simulink model "sm_tVtest_roller_idlerArm_i2u0l3"  (R2026a)
settings: Solver=VariableStepAuto  AbsTol=1e-3  EnableMultiTasking=on
undefined symbols (not defined in the file): P1, P2, P3, P4, P5, X, Y, Z
libraries: sm_lib x5, sm_trackV_lib_terrain_contact_elem x5, fl_lib x2, nesl_utility x2, sm_trackV_lib_chain_underc_elem x1, simulink x1, sm_rollerV_lib_underc_elem x1, sm_rollerV_lib_underc_idlerArm_i2u0l3 x1
Description:
  | Copyright 2024-2026 The MathWorks, Inc.
settings Model: Creator=smiller  LastModifiedBy=smiller
settings DebuggingCC: SubsystemReferenceDiagnosticForUnitTest=warning
settings SimscapeCC: SimscapeNominalValues="[{\"value\":\"1\",\"unit\":\"A\"},{\"value\":\"1\",\"unit\":\"bar\"},{\"value\":\"1\",\"unit\":\"cm^2\"},{\"value\":\"1\",\"unit\":\"cm^3/s\"},{\"value\":\"1\",\"unit\":\"kJ/kg\"},{\"value\":\"1\",\"unit\":\"kW\"},{\"value\":\"1\",\"unit\":\"l\"},{\"value\":\"1\",\"unit\":\"N\"},{\"value\":\"1\",\"unit\":\"N*m\"},{\"value\":\"1\",\"unit\":\"V\"}]"  SimscapeLogSimulationStatistics=on
settings DiagnosticsConfigSet: SimMechanicsUnconnectedFramePorts=none
settings ExplorerConfigSet: InternalSimMechanicsExplorerSettings="<ExplorerConfiguration><canonicalview>default</canonicalview><AnimationSetting><BasePlaybackSpeed>1.0</BasePlaybackSpeed><PlaybackSpeedFactor>1.0</PlaybackSpeedFactor></AnimationSetting><TilePanel><TileInfo><Tiles Columns=\"1\" Count=\"1\" Rows=\"1\"><Column Weight=\"1\"/><Row Weight=\"1\"/><Tile Height=\"1\" Width=\"1\" X=\"0\" Y=\"0\"/></Tiles></TileInfo><SceneInfo><SceneViewer><BGColor><R>1</R><G>1</G><B>1</B></BGColor><Camera><DoPerspective>off</DoPerspective><Position><X>0.567898563386482147</X><Y>-1.86694805060514923</Y><Z>1.30068286552298851</Z></Position><Center><X>0.185623686788384534</X><Y>-0.0132287901313050682</Y><Z>1.03548068078574151</Z></Center><Up><X>-0.02328869963817011</X><Y>0.136876623335939085</Y><Z>0.990314306901255881</Z></Up><ViewLimDist>1</ViewLimDist><YLim>1.16506449341773988</YLim><XLim>2.52473886880948983</XLim></Camera></SceneViewer></SceneInfo></TilePanel><MechEditorPanel><Cameras/><GfxPanelCameraMap/><VideoCreator><PlaybackSpeedRatio>1.0</PlaybackSpeedRatio><FrameRate>30</FrameRate><VideoFormat>Motion JPEG AVI</VideoFormat><FrameSize>auto</FrameSize></VideoCreator></MechEditorPanel></ExplorerConfiguration>"

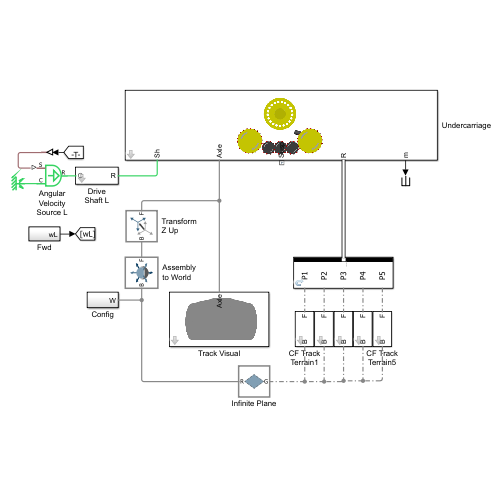
[thumbnail: Simulink's stored preview of the top-level diagram]
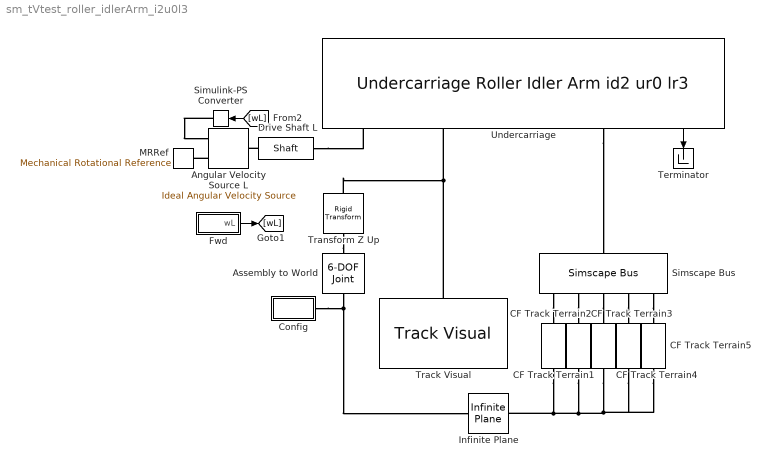
== system sm_tVtest_roller_idlerArm_i2u0l3 ==
  Angular Velocity Source L : fl_lib/Mechanical/Mechanical Sources/Ideal Angular Velocity Source
  Assembly to World : sm_lib/Joints/6-DOF Joint  JointMode=Normal  CompositeWrenchDir=FollowerOnBase  CompositeWrenchFrame=BaseFrame  SenseConstraintForce=off  SenseConstraintTorque=off  SenseTotalForce=off  SenseTotalTorque=off  PxPositionTargetSpecify=off  PxPositionTargetPriority=High  PxPositionTargetValue=0  PxPositionTargetValueUnits=m  PxVelocityTargetSpecify=off  PxVelocityTargetPriority=High  PxVelocityTargetValue=0  PxVelocityTargetValueUnits=m/s  PxEquilibriumPosition=0  PxEquilibriumPositionUnits=m  PxSpringStiffness=0  PxSpringStiffnessUnits=N/m  PxDampingCoefficient=0  PxDampingCoefficientUnits=N/(m/s)  PxLowerLimitSpecify=off  PxLowerLimitBound=-1  PxLowerLimitBoundUnits=m  PxLowerLimitStiffness=1e6  PxLowerLimitStiffnessUnits=N/m  PxLowerLimitDamping=1e3  PxLowerLimitDampingUnits=N/(m/s)  PxLowerLimitTransitionRegionWidth=1e-4  PxLowerLimitTransitionRegionWidthUnits=m  PxUpperLimitSpecify=off  PxUpperLimitBound=1  PxUpperLimitBoundUnits=m  PxUpperLimitStiffness=1e6  PxUpperLimitStiffnessUnits=N/m  PxUpperLimitDamping=1e3  PxUpperLimitDampingUnits=N/(m/s)  PxUpperLimitTransitionRegionWidth=1e-4  PxUpperLimitTransitionRegionWidthUnits=m  PxTorqueActuationMode=NoTorque  PxMotionActuationMode=ComputedMotion  PxSensePosition=off  PxSenseVelocity=off  PxSenseAcceleration=off  PxSenseTorqueForce=off  PxSenseLowerLimitTorqueForce=off  PxSenseUpperLimitTorqueForce=off  PyPositionTargetSpecify=off  PyPositionTargetPriority=High  PyPositionTargetValue=0  PyPositionTargetValueUnits=m  PyVelocityTargetSpecify=off  PyVelocityTargetPriority=High  PyVelocityTargetValue=0  PyVelocityTargetValueUnits=m/s  PyEquilibriumPosition=0  PyEquilibriumPositionUnits=m  PySpringStiffness=0  PySpringStiffnessUnits=N/m  PyDampingCoefficient=0  PyDampingCoefficientUnits=N/(m/s)  PyLowerLimitSpecify=off  PyLowerLimitBound=-1  PyLowerLimitBoundUnits=m  PyLowerLimitStiffness=1e6  PyLowerLimitStiffnessUnits=N/m  PyLowerLimitDamping=1e3  PyLowerLimitDampingUnits=N/(m/s)  PyLowerLimitTransitionRegionWidth=1e-4  PyLowerLimitTransitionRegionWidthUnits=m  PyUpperLimitSpecify=off  PyUpperLimitBound=1  PyUpperLimitBoundUnits=m  PyUpperLimitStiffness=1e6  PyUpperLimitStiffnessUnits=N/m  PyUpperLimitDamping=1e3  PyUpperLimitDampingUnits=N/(m/s)  PyUpperLimitTransitionRegionWidth=1e-4  PyUpperLimitTransitionRegionWidthUnits=m  PyTorqueActuationMode=NoTorque  PyMotionActuationMode=ComputedMotion  PySensePosition=off  PySenseVelocity=off  PySenseAcceleration=off  PySenseTorqueForce=off  PySenseLowerLimitTorqueForce=off  PySenseUpperLimitTorqueForce=off  PzPositionTargetSpecify=on  PzPositionTargetPriority=High  PzPositionTargetValue=1.5  PzPositionTargetValueUnits=m  PzVelocityTargetSpecify=off  PzVelocityTargetPriority=High  PzVelocityTargetValue=0  PzVelocityTargetValueUnits=m/s  PzEquilibriumPosition=0  PzEquilibriumPositionUnits=m  PzSpringStiffness=0  PzSpringStiffnessUnits=N/m  PzDampingCoefficient=0  PzDampingCoefficientUnits=N/(m/s)  PzLowerLimitSpecify=off  PzLowerLimitBound=-1  PzLowerLimitBoundUnits=m  PzLowerLimitStiffness=1e6  PzLowerLimitStiffnessUnits=N/m  PzLowerLimitDamping=1e3  PzLowerLimitDampingUnits=N/(m/s)  PzLowerLimitTransitionRegionWidth=1e-4  PzLowerLimitTransitionRegionWidthUnits=m  PzUpperLimitSpecify=off  PzUpperLimitBound=1  PzUpperLimitBoundUnits=m  PzUpperLimitStiffness=1e6  PzUpperLimitStiffnessUnits=N/m  PzUpperLimitDamping=1e3  PzUpperLimitDampingUnits=N/(m/s)  PzUpperLimitTransitionRegionWidth=1e-4  PzUpperLimitTransitionRegionWidthUnits=m  PzTorqueActuationMode=NoTorque  PzMotionActuationMode=ComputedMotion  PzSensePosition=off  PzSenseVelocity=off  PzSenseAcceleration=off  PzSenseTorqueForce=off  PzSenseLowerLimitTorqueForce=off  PzSenseUpperLimitTorqueForce=off  SphPositionTargetSpecify=off  SphPositionTargetPriority=High  SphPositionTargetRotationMethod=None  SphPositionTargetFollAlignAxisA=+X  SphPositionTargetBaseAlignAxisA=+Y  SphPositionTargetFollAlignAxisB=+Y  SphPositionTargetBaseAlignAxisB=+Z  SphPositionTargetRotationStandardAxis=+Z  SphPositionTargetRotationAngle=0.0  SphPositionTargetRotationAngleUnits=deg  SphPositionTargetRotationArbitraryAxis=[0 0 1]  SphPositionTargetRotationSequenceAxes=FollowerAxes  SphPositionTargetRotationSequence=XYX  SphPositionTargetRotationSequenceAngles=[0 0 0]  SphPositionTargetRotationSequenceAnglesUnits=deg  SphPositionTargetRotationMatrix=[1 0 0; 0 1 0; 0 0 1]  SphPositionTargetQuaternion=[1 0 0 0]  SphVelocityTargetSpecify=off  SphVelocityTargetPriority=High  SphVelocityTargetValue=[0 0 0]  SphVelocityTargetValueUnits=deg/s  SphVelocityTargetInFollowerFrame=on  SphEqPosRotationMethod=None  SphEqPosFollAlignAxisA=+X  SphEqPosBaseAlignAxisA=+Y  SphEqPosFollAlignAxisB=+Y  SphEqPosBaseAlignAxisB=+Z  SphEqPosRotationStandardAxis=+Z  SphEqPosRotationAngle=0.0  SphEqPosRotationAngleUnits=deg  SphEqPosRotationArbitraryAxis=[0 0 1]  SphEqPosRotationSequenceAxes=FollowerAxes  SphEqPosRotationSequence=XYX  SphEqPosRotationSequenceAngles=[0 0 0]  SphEqPosRotationSequenceAnglesUnits=deg  SphEqPosRotationMatrix=[1 0 0; 0 1 0; 0 0 1]  SphEqPosQuaternion=[1 0 0 0]  SphSpringStiffness=0  SphSpringStiffnessUnits=N*m/deg  SphDampingCoefficient=0  SphDampingCoefficientUnits=N*m/(deg/s)  SphLowerLimitSpecify=off  SphLowerLimitBound=15  SphLowerLimitBoundUnits=deg  SphLowerLimitStiffness=1e4  SphLowerLimitStiffnessUnits=N*m/deg  SphLowerLimitDamping=10  SphLowerLimitDampingUnits=N*m/(deg/s)  SphLowerLimitTransitionRegionWidth=0.1  SphLowerLimitTransitionRegionWidthUnits=deg  SphUpperLimitSpecify=off  SphUpperLimitBound=45  SphUpperLimitBoundUnits=deg  SphUpperLimitStiffness=1e4  SphUpperLimitStiffnessUnits=N*m/deg  SphUpperLimitDamping=10  SphUpperLimitDampingUnits=N*m/(deg/s)  SphUpperLimitTransitionRegionWidth=0.1  SphUpperLimitTransitionRegionWidthUnits=deg  SphTorqueActuationMode=NoTorque  SphActuateTorqueX=off  SphActuateTorqueY=off  SphActuateTorqueZ=off  SphActuateTorque=off  SphActuationFrame=BaseFrame  SphSensePosition=off  SphSenseVelocityX=off  SphSenseVelocityY=off  SphSenseVelocityZ=off  SphSenseVelocity=off  SphSenseAccelerationX=off  SphSenseAccelerationY=off  SphSenseAccelerationZ=off  SphSenseAcceleration=off  SphSenseLowerLimitTorqueMag=off  SphSenseUpperLimitTorqueMag=off  SphSensingFrame=BaseFrame
  CF Track Terrain{1..5} (5 alike) : sm_trackV_lib_terrain_contact_elem/CF Track Terrain  NormalStiffness=Scene.Contact.Terrain.K  NormalDamping=Scene.Contact.Terrain.B  NormalTransitionRegionWidth=Scene.Contact.Terrain.TW  CoefficientOfDynamicFriction=Scene.Contact.Terrain.mud  CoefficientOfStaticFriction=Scene.Contact.Terrain.mus  FrictionalCriticalVelocity=Scene.Contact.Terrain.CV
  Config : Subsystem
  Drive Shaft L : sm_trackV_lib_chain_underc_elem/Shaft  k_shaft=Excv.Drive.Shaft.k  b_shaft=Excv.Drive.Shaft.b
  Fwd : Subsystem  VariantControl=Fwd
  Infinite Plane : sm_lib/Curves and Surfaces/Infinite Plane  GraphicType=Rectangle  GraphicPlaneWidth=1  GraphicPlaneWidthUnits=m  GraphicPlaneHeight=1  GraphicPlaneHeightUnits=m  GraphicVisPropType=SimpleVisualProperties  GraphicDiffuseColor=[0.5 0.5 0.5]  GraphicOpacity=0.25  GraphicSpecularColor=[0.5 0.5 0.5 1.0]  GraphicAmbientColor=[0.15 0.15 0.15 1.0]  GraphicEmissiveColor=[0.0 0.0 0.0 1.0]  GraphicShininess=75
  MRRef : fl_lib/Mechanical/Rotational Elements/Mechanical Rotational Reference
  Simscape Bus : SimscapeBus  HierarchyStrings=P1;P2;P3;P4;P5  ConnectionType=Bus: CBO_Roller5
  Simulink-PS Converter : nesl_utility/Simulink-PS Converter  PhysicalDomain=network_engine_domain  SubClassName=ps_input  LeftPortType=input  RightPortType=output  PseudoPeriodic=off  Frequencies=[]  NoiseDistribution=none  NoiseParameters=[]  Unit=1  AffineConversion=off  FilteringAndDerivatives=provide  SimscapeFilterOrder=1  InputFilterTimeConstant=0.001  UdotUserProvided=0
  Terminator : Terminator
  Track Visual : sm_rollerV_lib_underc_elem/Track Visual  track_m=Trac.Vis.Track.m  track_cg_offset=Trac.Vis.Track.cg  track_axle_offset_x=Trac.Frame.SprkOffLon.Axle  track_axle_offset_y=Trac.Frame.SprkOffVer.Axle  track_moi=Trac.Vis.Track.moi  track_poi=Trac.Vis.Track.poi  track_xc=Trac.Vis.Track.track_xc  track_w=Trac.Belt.w  track_clr=Trac.Vis.Track.clr  track_opc=Trac.Vis.Track.opc
  Transform Z Up : sm_lib/Frames and Transforms/Rigid Transform  RotationMethod=StandardAxis  FollAlignAxisA=+X  BaseAlignAxisA=+Y  FollAlignAxisB=+Y  BaseAlignAxisB=+Z  RotationStandardAxis=+X  RotationAngle=-90  RotationAngleUnits=deg  RotationArbitraryAxis=[0 0 1]  RotationSequenceAxes=FollowerAxes  RotationSequence=XYX  RotationSequenceAngles=[0 0 0]  RotationSequenceAnglesUnits=deg  RotationMatrix=[1 0 0; 0 1 0; 0 0 1]  Quaternion=[1 0 0 0]  TranslationMethod=None  TranslationCartesianOffset=[0 0 0]  TranslationCartesianOffsetUnits=m  TranslationStandardAxis=+Z  TranslationStandardOffset=0  TranslationStandardOffsetUnits=m  TranslationROffset=0  TranslationROffsetUnits=m  TranslationThetaOffset=0  TranslationThetaOffsetUnits=deg  TranslationZOffset=0  TranslationZOffsetUnits=m
  Undercarriage : sm_rollerV_lib_underc_idlerArm_i2u0l3/Undercarriage Roller Idler Arm id2 ur0 lr3  popup_leftOrRight=Right  sprk_rad_roll=Trac.Sprocket.Roller.rad  sprk_wid_roll=Trac.Sprocket.Roller.wid  sprk_clr=Trac.Sprocket.Roller.clr  sprk_opc=Trac.Sprocket.Roller.opc  sprk_rim_ir=Trac.Sprocket.Rim.rad_inner  sprk_rim_thk=Trac.Sprocket.Rim.thk  sprk_rim_spoke_xc=Trac.Sprocket.Rim.spoke_xc  sprk_rad_pitch=Trac.Sprocket.Spoke.pitch_rad  sprk_spoke_rad=Trac.Sprocket.Spoke.rad  sprk_spoke_len=Trac.Sprocket.Spoke.len  sprk_spoke_num=Trac.Sprocket.nSpokes  idlerR_rad=Trac.IdlerR.rad  idlerF_rad=Trac.IdlerF.rad  idlerR_total_len=Trac.IdlerR.len_total  idlerF_total_len=Trac.IdlerF.len_total  idlerR_avg_rho=Trac.IdlerR.rho_avg  idlerF_avg_rho=Trac.IdlerF.rho_avg  idlerR_clr=Trac.IdlerR.clr  idlerF_clr=Trac.IdlerF.clr  idlerR_opc=Trac.IdlerR.opc  idlerF_opc=Trac.IdlerF.opc  idlerR_contgeo_ptcld=Trac.IdlerR.ground_contact.ptcld.pts  idlerF_contgeo_ptcld=Trac.IdlerF.ground_contact.ptcld.pts  idlerR_contgeo_rad=Trac.IdlerR.ground_contact.ptcld.rad  idlerF_contgeo_rad=Trac.IdlerF.ground_contact.ptcld.rad  idlerR_contgeo_clr=Trac.IdlerR.belt_contact.clr  idlerF_contgeo_clr=Trac.IdlerF.belt_contact.clr  idlerR_contgeo_opc=Trac.IdlerR.belt_contact.opc  idlerF_contgeo_opc=Trac.IdlerF.belt_contact.opc  arm_idlerc=Trac.IdlerArm.Pivot_to_Idler  arm_tens_x=Trac.IdlerArm.Pivot_to_TensionerX  arm_tens_y=Trac.IdlerArm.Pivot_to_TensionerY  arm_wid=Trac.IdlerArm.wid  arm_thk=Trac.IdlerArm.thk  arm_rho=Trac.IdlerArm.rho  arm_clr=Trac.IdlerArm.clr  arm_opc=Trac.IdlerArm.opc  roller_lower_len=Trac.Roller.Lower.len  roller_lower_rad=Trac.Roller.Lower.rad  roller_lower_rho=Trac.Roller.Lower.rho  roller_lower_clr=Trac.Roller.Lower.clr  roller_lower_opc=Trac.Roller.Lower.opc  roller_lower_contgeo_clr=Trac.Roller.Lower.belt_contact.clr  roller_lower_contgeo_opc=Trac.Roller.Lower.belt_contact.opc  roller_lower_contgeo_ptcld=Trac.Roller.Lower.ground_contact.ptcld.pts  roller_lower_contgeo_rad=Trac.Roller.Lower.ground_contact.ptcld.rad  tensioner_cyl_len=Trac.IdlerF.Tensioner.cyl.len  tensioner_cyl_rad=Trac.IdlerF.Tensioner.cyl.rad  tensioner_cyl_rho=Trac.IdlerF.Tensioner.cyl.rho  tensioner_cyl_clr=Trac.IdlerF.Tensioner.cyl.clr  tensioner_cyl_opc=Trac.IdlerF.Tensioner.cyl.opc  tensioner_pist_len=Trac.IdlerF.Tensioner.piston.len  tensioner_pist_rad=Trac.IdlerF.Tensioner.piston.rad  tensioner_pist_rho=Trac.IdlerF.Tensioner.piston.rho  tensioner_pist_clr=Trac.IdlerF.Tensioner.piston.clr  tensioner_pist_opc=Trac.IdlerF.Tensioner.piston.opc  tensioner_br_len=Trac.IdlerF.Tensioner.bracket.len  tensioner_br_width=Trac.IdlerF.Tensioner.bracket.wid  tensioner_br_height=Trac.IdlerF.Tensioner.bracket.height  tensioner_br_thk=Trac.IdlerF.Tensioner.bracket.thk  tensioner_br_rho=Trac.IdlerF.Tensioner.bracket.rho  tensioner_br_clr=Trac.IdlerF.Tensioner.bracket.clr  tensioner_br_opc=Trac.IdlerF.Tensioner.bracket.opc  tensioner_eqpos=Trac.IdlerF.Tensioner.xeq  tensioner_x0=Trac.IdlerF.Tensioner.x0  tensioner_k=Trac.IdlerF.Tensioner.K  tensioner_b=Trac.IdlerF.Tensioner.B  popup_trackFrame=Fixed  roller_lower_x=Trac.Frame.SprkOffLon.Lower  axle_x=Trac.Frame.SprkOffLon.Axle  idlerFix_x=Trac.Frame.SprkOffLon.IdlerR  frame_pivot_x=Trac.Frame.SprkOffLon.PivotFra  tensionC_x=Trac.Frame.SprkOffLon.TensionC  idlerArm_x=Trac.Frame.SprkOffLon.IdlerArm  roller_lower_y=Trac.Frame.SprkOffVer.Lower  axle_y=Trac.Frame.SprkOffVer.Axle  idlerArm_y=Trac.Frame.SprkOffVer.IdlerArm  idlerFix_y=Trac.Frame.SprkOffVer.IdlerR  frame_pivot_y=Trac.Frame.SprkOffVer.PivotFra  tensionC_y=Trac.Frame.SprkOffVer.TensionC  frame_cg_offset=Trac.Frame.TrackFrame.CG  frame_mass=Trac.Frame.TrackFrame.Mass  frame_moi=Trac.Frame.TrackFrame.MOI  frame_poi=Trac.Frame.TrackFrame.POI  frame_roller_cg_offset=Trac.Frame.SprkFrame.CG  frame_roller_mass=Trac.Frame.SprkFrame.Mass  frame_roller_moi=Trac.Frame.SprkFrame.MOI  frame_roller_poi=Trac.Frame.SprkFrame.POI  frame_susp_offset=Trac.Frame.SuspOffset  roller_frame_pivot_range=Trac.Frame.PivotFra.Range  roller_frame_pivot_k=Trac.Frame.PivotFra.LimitK  roller_frame_pivot_b=Trac.Frame.PivotFra.LimitB  roller_frame_pivot_tw=Trac.Frame.PivotFra.LimitTW  sprk_rolling_rad=Trac.Sprocket.ground_contact.rolling_radius  roller_lower_rolling_rad=Trac.Roller.Lower.ground_contact.rolling_radius  idlerF_rolling_rad=Trac.IdlerF.ground_contact.rolling_radius  idlerR_rolling_rad=Trac.IdlerR.ground_contact.rolling_radius  rolling_cyl_len=Trac.Belt.w  accent_vis_lext=1e-3  roller_lower_cyl_clr=Trac.Roller.Lower.clr  roller_lower_cyl_opc=Trac.Roller.Lower.opc  idlerR_rollvervis_clr=Trac.IdlerR.clr  idlerF_rollvervis_clr=Trac.IdlerF.clr  idlerR_rollervis_opc=Trac.IdlerR.opc  idlerF_rollervis_opc=Trac.IdlerF.opc  accMn=0.65  accMx=0.75  acc_clr=[0.8 0.8 0.8]  acc_opc=1  popup_sense_roller=Actuator Torque
  wires:
  Fwd/1(wL) -> [wL]
  [wL] -> Simulink-PS Converter/1
  Undercarriage/1 -> Terminator/1
  connections:
  Angular Velocity Source L/RConn2 -- MRRef/LConn1
  Simulink-PS Converter/RConn1 -- Angular Velocity Source L/RConn1
  Drive Shaft L/LConn1 -- Angular Velocity Source L/LConn1
  Drive Shaft L/RConn1 -- Undercarriage/RConn4
  Undercarriage/RConn1 -- Simscape Bus/RConn1
  Transform Z Up/RConn1 -- Undercarriage/RConn3 -- Track Visual/LConn1
  CF Track Terrain2/LConn1 -- CF Track Terrain5/LConn1 -- CF Track Terrain4/LConn1 -- CF Track Terrain3/LConn1 -- CF Track Terrain1/LConn1 -- Infinite Plane/RConn1
  Simscape Bus/LConn1 -- CF Track Terrain1/RConn1
  Simscape Bus/LConn2 -- CF Track Terrain2/RConn1
  Simscape Bus/LConn3 -- CF Track Terrain3/RConn1
  Simscape Bus/LConn4 -- CF Track Terrain4/RConn1
  Simscape Bus/LConn5 -- CF Track Terrain5/RConn1
  Transform Z Up/LConn1 -- Assembly to World/RConn1
  Assembly to World/LConn1 -- Infinite Plane/LConn1 -- Config/RConn1

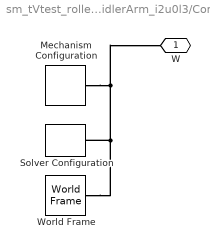
== system sm_tVtest_roller_idlerArm_i2u0l3/Config ==
  Mechanism Configuration : sm_lib/Utilities/Mechanism Configuration  UniformGravity=Constant  GravityVector=[0 0 -9.80665]  GravityVectorUnits=m/s^2  LinearizationDelta=0.001  JointModeTransitionNonlinearIterations=2
  Solver Configuration : nesl_utility/Solver Configuration  PhysicalDomain=network_engine_domain  SubClassName=solver  LeftPortType=input  RightPortType=generic  Tones=[]  Harmonics=[]  SimulateNoise=off  Profile=off  UseLocalSampling=off  EnableSwitchedLinearOptims=on  FrequencyDomain=off  UseCCode=off  RelTol=0.001  AbsTol=1e-06  MinStep=1e-09  ToWorkspace=off  RevertToSquareIcSolve=off  NumHomotopyIterations=100  PhasorMode=off  PhasorModeNumHarmonics=1  ConsistencySolver=NEWTON_XTOL_AFTER_FTOL  CanonicalOrdering=UNORDERED  OptimizeIntermediates=UNOPTIMIZED  IndexReductionMethod=DerivativeReplacement  DoDC=off  ResidualTolerance=1e-09  ConsistencyTolSource=GLOBAL  ConsistencyAbsTol=0.001  ConsistencyRelTol=0.001  ConsistencyTolFactor=0.001  UseLocalSolver=off  LocalSolverChoice=NE_BACKWARD_EULER_ADVANCER  ResolveIndetEquations=on  FunctionEvalNumThread=1  LocalSolverSampleTime=0.001  DoFixedCost=off  MaxNonlinIter=3  MaxModeIter=2  ComputeImpulses=off  ImpulseIterations=2  LinearAlgebra=Sparse  LinearAlgebraNumThread=0  EquationFormulation=NE_TIME_EF  DelaysMemoryBudget=1024  AutomaticFiltering=on  FilteringTimeConstant=0.001  PartitionStorageMethod=AS_NEEDED  PartitionMemoryBudget=1024  PartitionMethod=FAST  MultibodyUseLocalSolver=off  MultibodyLocalSolverChoice=ODE1  MultibodyLocalSolverSampleTime=0.001
  World Frame : sm_lib/Frames and Transforms/World Frame
  W : PMIOPort  Side=Right
  connections:
  World Frame/RConn1 -- W/RConn1 -- Mechanism Configuration/RConn1 -- Solver Configuration/RConn1

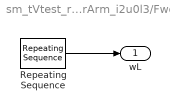
== system sm_tVtest_roller_idlerArm_i2u0l3/Fwd ==
  Repeating Sequence : simulink/Sources/Repeating Sequence  rep_seq_t=[0 2 2.01 40]  rep_seq_y=[0 0 3 3]
  wL : Outport
  wires:
  Repeating Sequence/1 -> wL/1
